simulink model "Non_WindFarm"  (R2024a)
settings: Solver=ode45  StartTime=parSimulacio.ti  StopTime=200  MaxStep=parSimulacio.pas  RelTol=1e-6  AbsTol=1e-6  EnableMultiTasking=on
model workspace (MAT data in the model file):
  tt_vw : Simulink.Parameter (value not decoded)
values from neighbouring files (symbols this model uses):
  L = L'    [Lin_SignalGenerator.m]    (also in Non_ParameterInitialize.m; cal_QR.m = zeros(v, 1); parameters_windFarm2.m)
  nu = size(S, 1)    [Lin_SignalGenerator.m]    (also in Non_ParameterInitialize.m; parameters_windFarm2.m)
  S = zeros(v, v)    [cal_QR.m]
  w0 = [1 -0.00962521549583 0.0254779042049 -0.0160197396127 -0.0156056332727 0.0112137208272 0.0440607583301 -0.0193704893312 -0.0229464276306 -0.00247675309015 0.0285830611299]    [w0.mat]
undefined symbols (not defined in the file or in its folder): parControl, parConvertidor, parGenerador, parGrid, parMecanica, parSimulacio, windspeed
(part 10 of 40)

== system Non_WindFarm/FOM/Wind Farm/Wind Turbine Strings/String6/WT3/WFG ==
  note: input output sign
  note: WE
  note: generator shaft angle
  note: generator speed
  vcqd : Inport
  Bus Continua1 : Subsystem  mask{tempPar=parConvertidor}
      mask prompts: tempPar "Estruc. Parametres"
      mask init:
      | C=tempPar.C;
      | E0=tempPar.E0;
  Clock : Clock
  Constant2 : Constant  Value=10
  Control Electric Generador : Subsystem  mask{tempPar=parControl.Electric.Generador}
      mask prompts: tempPar "Estruc. Parametres"
      mask init: same as Non_WindFarm/FOM/Wind Farm/Wind Turbine Strings/String1/WT1/WFG/Control Electric Generador
  Control Electric Tensio : Subsystem  mask{tempPar=parControl.Electric.BusContinua}
      mask prompts: tempPar "Estruc. Parametres"
      mask init:
      | Kp=tempPar.Kp;
      | Ki=tempPar.Ki;
      | Easterisc=tempPar.Easterisc;
  Control Mecanic : Subsystem  mask{tempPar=parControl.Mecanic}
      mask prompts: tempPar "Escruc. Parametres"
      mask init:
      | %Kp=tempPar.Kp;
      | T=tempPar.T;
      | KCP=tempPar.KCP;
      | omegamn=tempPar.omegamn;
      | Kp=tempPar.Kp;
      | Ki=tempPar.Ki;
  Control de Corrent de Xarxa2 : Subsystem  mask{tempPar=parControl.Electric.BandaXarxa}
      mask prompts: tempPar "Estruc. Parametres"
      mask init:
      | Kp=tempPar.Kp;
      | Ki=tempPar.Ki;
      | Ll=tempPar.Ll;
      | rl=tempPar.rl;
  Filtre de Xarxa1 : Subsystem  mask{tempPar=parConvertidor}
      mask prompts: tempPar "Estruc. Parametres"
      mask init:
      | rl=tempPar.rl;
      | Ll=tempPar.Ll;
  Gain : Gain  Gain=-1
  Maquina Sincrona : Subsystem  mask{tempPar=parGenerador}
      mask prompts: tempPar "Estruct. Parametres"
      mask init:
      | rs=tempPar.rs;
      | Lq=tempPar.Lq;
      | Ld=tempPar.Ld;
      | lambda_m=tempPar.lambda_m;
      | P=tempPar.P;
      | isqd0=tempPar.isqd0;
  Mecanica nolineal i vent : Subsystem  mask{tempPar=parMecanica}
      mask prompts: tempPar "Estruc. Parametres"
      mask init: same as Non_WindFarm/FOM/Wind Farm/Wind Turbine Strings/String1/WT1/WFG/Mecanica nolineal i vent
  Park : Subsystem
  Product1 : Product  Multiplication=Matrix(*)  RndMeth=Zero
  Product4 : Product  Multiplication=Matrix(*)  RndMeth=Zero
  Scope : Scope
  we : Gain  Gain=100*pi
  wind speed : Constant  Value=windspeed.string2
  ilqd : Outport
  wires:
  Mecanica nolineal i vent/1(omega_m) -> Control Electric Generador/4(omega_m), Control Mecanic/1(omega_m), Maquina Sincrona/2(omega_m)
  Mecanica nolineal i vent/2(theta_m) -> Maquina Sincrona/3(theta_m), Control Electric Generador/5(theta_m)
  Maquina Sincrona/2(parell_m) -> Mecanica nolineal i vent/1(parell_m)
  Control de Corrent de Xarxa2/1(vlabc) -> Bus Continua1/2(vlabc), Filtre de Xarxa1/2(vlabc)
  Bus Continua1/1(E) -> Control Electric Tensio/1(E), Control de Corrent de Xarxa2/4(E)
  Maquina Sincrona/1(isabc) -> Bus Continua1/4(isabc), Control Electric Generador/3(isabc)
  Control Electric Generador/1(vscabc) -> Bus Continua1/3(vsabc), Maquina Sincrona/1(vsabc)
  Filtre de Xarxa1/1(ilabc) -> Bus Continua1/1(ilabc), Product1/2, Control de Corrent de Xarxa2/2(ilabc)
  Bus Continua1/2(iDCm) -> Control Electric Tensio/2(IDCm)
  wind speed/1 -> Mecanica nolineal i vent/3(vw)
  Control Electric Tensio/1(iDCla) -> Control de Corrent de Xarxa2/3(iDCla)
  Constant2/1 -> Control Electric Generador/2(Q_sa)
  Control Mecanic/2(theta_a) -> Mecanica nolineal i vent/2(theta_a)
  Park/2(nTthetar) -> Product4/1
  vcqd/1 -> Product4/2
  Product4/1 -> Scope/1, Control de Corrent de Xarxa2/1(vzabc), Filtre de Xarxa1/1(vzabc)
  Park/1(Tthetar) -> Product1/1
  Clock/1 -> we/1
  we/1 -> Park/1(theta_r)
  Gain/1 -> ilqd/1
  Product1/1 -> Gain/1
  Control Mecanic/1(parell_ma) -> Control Electric Generador/1(parell_ma)

== system Non_WindFarm/FOM/Wind Farm/Wind Turbine Strings/String6/WT4/C_cable ==
  note: Vc_cable
  It2 : Inport
  I_in : Inport  Port=2
  I_cable : Inport  Port=3
  Add : Sum  Inputs=++-
  produce Vc_cable : StateSpace  A=[0,-100*pi;100*pi,0]  B=eye(2)/parGrid.WTstring.C_cable  C=eye(2)  D=zeros(2,2)  InitialCondition=sqrt(2)*66000/sqrt(3)*[1;0]
  Vc_cable : Outport
  wires:
  produce Vc_cable/1 -> Vc_cable/1
  Add/1 -> produce Vc_cable/1
  It2/1 -> Add/1
  I_cable/1 -> Add/3
  I_in/1 -> Add/2

== system Non_WindFarm/FOM/Wind Farm/Wind Turbine Strings/String6/WT4/C_filter ==
  note: Vc_filter
  IWF : Inport
  It1 : Inport  Port=2
  Add : Sum  Inputs=+-
  produce Vc_filter : StateSpace  A=[0,-100*pi;100*pi,0]  B=eye(2)/parConvertidor.Cfilt  C=eye(2)  D=zeros(2,2)  InitialCondition=sqrt(2)*970/sqrt(3)*[1;0]
  Vc_filter_qd : Outport
  wires:
  IWF/1 -> Add/1
  It1/1 -> Add/2
  Add/1 -> produce Vc_filter/1
  produce Vc_filter/1 -> Vc_filter_qd/1

== system Non_WindFarm/FOM/Wind Farm/Wind Turbine Strings/String6/WT4/Cable line ==
  V : Inport
  Vc_cable : Inport  Port=2
  1/L_Cable : Gain  Gain=1/parGrid.WTstring.Lcable
  A : Constant  Value=[parGrid.WTstring.rcable,100*pi*parGrid.WTstring.Lcable;-100*pi*parGrid.WTstring.Lcable,parGrid.WTstring.rcable]
  Add : Sum  Inputs=+--
  Integrator : Integrator
  Product6 : Product  Multiplication=Matrix(*)
  I_cable : Outport
  wires:
  Integrator/1 -> Product6/2, I_cable/1
  Vc_cable/1 -> Add/1
  V/1 -> Add/2
  A/1 -> Product6/1
  Product6/1 -> Add/3
  1/L_Cable/1 -> Integrator/1
  Add/1 -> 1/L_Cable/1

== system Non_WindFarm/FOM/Wind Farm/Wind Turbine Strings/String6/WT4/Transformer-complex ==
  note: It1
  note: Vt1
  Vc_filter_qd : Inport
  Vc_cable_qd : Inport  Port=2
  1/(N1N2) : Gain  Gain=1/parGrid.N1N2
  1/(N1N2)1 : Gain  Gain=1/parGrid.N1N2
  1/[Lt+Lt1/(N1N2^2)] : Gain  Gain=1/(parGrid.WTtransf.Lt+parGrid.WTtransf.Lt2/(parGrid.N1N2^2))
  Add4 : Sum  Inputs=-+-
  Integrator2 : Integrator
  Product6 : Product  Multiplication=Matrix(*)
  "[A+A1/(N1N2^2)]" : Constant  Value=[parGrid.WTtransf.rt,100*pi*parGrid.WTtransf.Lt;-100*pi*parGrid.WTtransf.Lt,parGrid.WTtransf.rt]+[parGrid.WTtransf.rt2,100*pi*parGrid.WTtransf.Lt2;-100*pi*parGrid.WTtransf.Lt2,parGrid.WTtransf.rt2]/(parGrid.N1N2^2)
  homopolar sequence : Subsystem  Commented=through
  It1 : Outport
  It2 : Outport  Port=2
  wires:
  Vc_cable_qd/1 -> homopolar sequence/1(Vc_cable_qd)
  Add4/1 -> 1/[Lt+Lt1/(N1N2^2)]/1
  1/(N1N2)/1 -> Add4/1
  Vc_filter_qd/1 -> homopolar sequence/2(Vc_filter_qd)
  Product6/1 -> Add4/3
  Integrator2/1 -> Product6/2, It1/1, 1/(N1N2)1/1
  1/(N1N2)1/1 -> It2/1
  1/[Lt+Lt1/(N1N2^2)]/1 -> Integrator2/1
  homopolar sequence/1(Vc_cable_bar) -> 1/(N1N2)/1
  homopolar sequence/2(Vc_filter_bar) -> Add4/2
  "[A+A1/(N1N2^2)]"/1 -> Product6/1

== system Non_WindFarm/FOM/Wind Farm/Wind Turbine Strings/String6/WT4/WFG ==
  note: input output sign
  note: WE
  note: generator shaft angle
  note: generator speed
  vcqd : Inport
  Bus Continua1 : Subsystem  mask{tempPar=parConvertidor}
      mask prompts: tempPar "Estruc. Parametres"
      mask init:
      | C=tempPar.C;
      | E0=tempPar.E0;
  Clock : Clock
  Constant2 : Constant  Value=10
  Control Electric Generador : Subsystem  mask{tempPar=parControl.Electric.Generador}
      mask prompts: tempPar "Estruc. Parametres"
      mask init: same as Non_WindFarm/FOM/Wind Farm/Wind Turbine Strings/String1/WT1/WFG/Control Electric Generador
  Control Electric Tensio : Subsystem  mask{tempPar=parControl.Electric.BusContinua}
      mask prompts: tempPar "Estruc. Parametres"
      mask init:
      | Kp=tempPar.Kp;
      | Ki=tempPar.Ki;
      | Easterisc=tempPar.Easterisc;
  Control Mecanic : Subsystem  mask{tempPar=parControl.Mecanic}
      mask prompts: tempPar "Escruc. Parametres"
      mask init:
      | %Kp=tempPar.Kp;
      | T=tempPar.T;
      | KCP=tempPar.KCP;
      | omegamn=tempPar.omegamn;
      | Kp=tempPar.Kp;
      | Ki=tempPar.Ki;
  Control de Corrent de Xarxa2 : Subsystem  mask{tempPar=parControl.Electric.BandaXarxa}
      mask prompts: tempPar "Estruc. Parametres"
      mask init:
      | Kp=tempPar.Kp;
      | Ki=tempPar.Ki;
      | Ll=tempPar.Ll;
      | rl=tempPar.rl;
  Filtre de Xarxa1 : Subsystem  mask{tempPar=parConvertidor}
      mask prompts: tempPar "Estruc. Parametres"
      mask init:
      | rl=tempPar.rl;
      | Ll=tempPar.Ll;
  Gain : Gain  Gain=-1
  Maquina Sincrona : Subsystem  mask{tempPar=parGenerador}
      mask prompts: tempPar "Estruct. Parametres"
      mask init:
      | rs=tempPar.rs;
      | Lq=tempPar.Lq;
      | Ld=tempPar.Ld;
      | lambda_m=tempPar.lambda_m;
      | P=tempPar.P;
      | isqd0=tempPar.isqd0;
  Mecanica nolineal i vent : Subsystem  mask{tempPar=parMecanica}
      mask prompts: tempPar "Estruc. Parametres"
      mask init: same as Non_WindFarm/FOM/Wind Farm/Wind Turbine Strings/String1/WT1/WFG/Mecanica nolineal i vent
  Park : Subsystem
  Product1 : Product  Multiplication=Matrix(*)  RndMeth=Zero
  Product4 : Product  Multiplication=Matrix(*)  RndMeth=Zero
  Scope : Scope
  we : Gain  Gain=100*pi
  wind speed : Constant  Value=windspeed.string2
  ilqd : Outport
  wires:
  Mecanica nolineal i vent/1(omega_m) -> Control Electric Generador/4(omega_m), Control Mecanic/1(omega_m), Maquina Sincrona/2(omega_m)
  Mecanica nolineal i vent/2(theta_m) -> Maquina Sincrona/3(theta_m), Control Electric Generador/5(theta_m)
  Maquina Sincrona/2(parell_m) -> Mecanica nolineal i vent/1(parell_m)
  Control de Corrent de Xarxa2/1(vlabc) -> Bus Continua1/2(vlabc), Filtre de Xarxa1/2(vlabc)
  Bus Continua1/1(E) -> Control Electric Tensio/1(E), Control de Corrent de Xarxa2/4(E)
  Maquina Sincrona/1(isabc) -> Bus Continua1/4(isabc), Control Electric Generador/3(isabc)
  Control Electric Generador/1(vscabc) -> Bus Continua1/3(vsabc), Maquina Sincrona/1(vsabc)
  Filtre de Xarxa1/1(ilabc) -> Bus Continua1/1(ilabc), Product1/2, Control de Corrent de Xarxa2/2(ilabc)
  Bus Continua1/2(iDCm) -> Control Electric Tensio/2(IDCm)
  wind speed/1 -> Mecanica nolineal i vent/3(vw)
  Control Electric Tensio/1(iDCla) -> Control de Corrent de Xarxa2/3(iDCla)
  Constant2/1 -> Control Electric Generador/2(Q_sa)
  Control Mecanic/2(theta_a) -> Mecanica nolineal i vent/2(theta_a)
  Park/2(nTthetar) -> Product4/1
  vcqd/1 -> Product4/2
  Product4/1 -> Scope/1, Control de Corrent de Xarxa2/1(vzabc), Filtre de Xarxa1/1(vzabc)
  Park/1(Tthetar) -> Product1/1
  Clock/1 -> we/1
  we/1 -> Park/1(theta_r)
  Gain/1 -> ilqd/1
  Product1/1 -> Gain/1
  Control Mecanic/1(parell_ma) -> Control Electric Generador/1(parell_ma)

== system Non_WindFarm/FOM/Wind Farm/Wind Turbine Strings/String6/WT5/C_cable ==
  note: Vc_cable
  It2 : Inport
  I_in : Inport  Port=2
  I_cable : Inport  Port=3
  Add : Sum  Inputs=++-
  produce Vc_cable : StateSpace  A=[0,-100*pi;100*pi,0]  B=eye(2)/parGrid.WTstring.C_cable  C=eye(2)  D=zeros(2,2)  InitialCondition=sqrt(2)*66000/sqrt(3)*[1;0]
  Vc_cable : Outport
  wires:
  I_in/1 -> Add/2
  I_cable/1 -> Add/3
  It2/1 -> Add/1
  Add/1 -> produce Vc_cable/1
  produce Vc_cable/1 -> Vc_cable/1

== system Non_WindFarm/FOM/Wind Farm/Wind Turbine Strings/String6/WT5/C_filter ==
  note: Vc_filter
  IWF : Inport
  It1 : Inport  Port=2
  Add : Sum  Inputs=+-
  produce Vc_filter : StateSpace  A=[0,-100*pi;100*pi,0]  B=eye(2)/parConvertidor.Cfilt  C=eye(2)  D=zeros(2,2)  InitialCondition=sqrt(2)*970/sqrt(3)*[1;0]
  Vc_filter_qd : Outport
  wires:
  produce Vc_filter/1 -> Vc_filter_qd/1
  Add/1 -> produce Vc_filter/1
  It1/1 -> Add/2
  IWF/1 -> Add/1

== system Non_WindFarm/FOM/Wind Farm/Wind Turbine Strings/String6/WT5/Cable line ==
  V : Inport
  Vc_cable : Inport  Port=2
  1/L_Cable : Gain  Gain=1/parGrid.WTstring.Lcable
  A : Constant  Value=[parGrid.WTstring.rcable,100*pi*parGrid.WTstring.Lcable;-100*pi*parGrid.WTstring.Lcable,parGrid.WTstring.rcable]
  Add : Sum  Inputs=+--
  Integrator : Integrator
  Product6 : Product  Multiplication=Matrix(*)
  I_cable : Outport
  wires:
  Add/1 -> 1/L_Cable/1
  1/L_Cable/1 -> Integrator/1
  Product6/1 -> Add/3
  A/1 -> Product6/1
  V/1 -> Add/2
  Vc_cable/1 -> Add/1
  Integrator/1 -> I_cable/1, Product6/2

== system Non_WindFarm/FOM/Wind Farm/Wind Turbine Strings/String6/WT5/Transformer-complex ==
  note: Vt1
  note: It1
  Vc_filter_qd : Inport
  Vc_cable_qd : Inport  Port=2
  1/(N1N2) : Gain  Gain=1/parGrid.N1N2
  1/(N1N2)1 : Gain  Gain=1/parGrid.N1N2
  1/[Lt+Lt1/(N1N2^2)] : Gain  Gain=1/(parGrid.WTtransf.Lt+parGrid.WTtransf.Lt2/(parGrid.N1N2^2))
  Add4 : Sum  Inputs=-+-
  Integrator2 : Integrator
  Product6 : Product  Multiplication=Matrix(*)
  "[A+A1/(N1N2^2)]" : Constant  Value=[parGrid.WTtransf.rt,100*pi*parGrid.WTtransf.Lt;-100*pi*parGrid.WTtransf.Lt,parGrid.WTtransf.rt]+[parGrid.WTtransf.rt2,100*pi*parGrid.WTtransf.Lt2;-100*pi*parGrid.WTtransf.Lt2,parGrid.WTtransf.rt2]/(parGrid.N1N2^2)
  homopolar sequence : Subsystem  Commented=through
  It1 : Outport
  It2 : Outport  Port=2
  wires:
  "[A+A1/(N1N2^2)]"/1 -> Product6/1
  homopolar sequence/2(Vc_filter_bar) -> Add4/2
  homopolar sequence/1(Vc_cable_bar) -> 1/(N1N2)/1
  1/[Lt+Lt1/(N1N2^2)]/1 -> Integrator2/1
  1/(N1N2)1/1 -> It2/1
  Integrator2/1 -> 1/(N1N2)1/1, It1/1, Product6/2
  Product6/1 -> Add4/3
  Vc_filter_qd/1 -> homopolar sequence/2(Vc_filter_qd)
  1/(N1N2)/1 -> Add4/1
  Add4/1 -> 1/[Lt+Lt1/(N1N2^2)]/1
  Vc_cable_qd/1 -> homopolar sequence/1(Vc_cable_qd)

== system Non_WindFarm/FOM/Wind Farm/Wind Turbine Strings/String6/WT5/WFG ==
  note: input output sign
  note: WE
  note: generator shaft angle
  note: generator speed
  vcqd : Inport
  Bus Continua1 : Subsystem  mask{tempPar=parConvertidor}
      mask prompts: tempPar "Estruc. Parametres"
      mask init:
      | C=tempPar.C;
      | E0=tempPar.E0;
  Clock : Clock
  Constant2 : Constant  Value=10
  Control Electric Generador : Subsystem  mask{tempPar=parControl.Electric.Generador}
      mask prompts: tempPar "Estruc. Parametres"
      mask init: same as Non_WindFarm/FOM/Wind Farm/Wind Turbine Strings/String1/WT1/WFG/Control Electric Generador
  Control Electric Tensio : Subsystem  mask{tempPar=parControl.Electric.BusContinua}
      mask prompts: tempPar "Estruc. Parametres"
      mask init:
      | Kp=tempPar.Kp;
      | Ki=tempPar.Ki;
      | Easterisc=tempPar.Easterisc;
  Control Mecanic : Subsystem  mask{tempPar=parControl.Mecanic}
      mask prompts: tempPar "Escruc. Parametres"
      mask init:
      | %Kp=tempPar.Kp;
      | T=tempPar.T;
      | KCP=tempPar.KCP;
      | omegamn=tempPar.omegamn;
      | Kp=tempPar.Kp;
      | Ki=tempPar.Ki;
  Control de Corrent de Xarxa2 : Subsystem  mask{tempPar=parControl.Electric.BandaXarxa}
      mask prompts: tempPar "Estruc. Parametres"
      mask init:
      | Kp=tempPar.Kp;
      | Ki=tempPar.Ki;
      | Ll=tempPar.Ll;
      | rl=tempPar.rl;
  Filtre de Xarxa1 : Subsystem  mask{tempPar=parConvertidor}
      mask prompts: tempPar "Estruc. Parametres"
      mask init:
      | rl=tempPar.rl;
      | Ll=tempPar.Ll;
  Gain : Gain  Gain=-1
  Maquina Sincrona : Subsystem  mask{tempPar=parGenerador}
      mask prompts: tempPar "Estruct. Parametres"
      mask init:
      | rs=tempPar.rs;
      | Lq=tempPar.Lq;
      | Ld=tempPar.Ld;
      | lambda_m=tempPar.lambda_m;
      | P=tempPar.P;
      | isqd0=tempPar.isqd0;
  Mecanica nolineal i vent : Subsystem  mask{tempPar=parMecanica}
      mask prompts: tempPar "Estruc. Parametres"
      mask init: same as Non_WindFarm/FOM/Wind Farm/Wind Turbine Strings/String1/WT1/WFG/Mecanica nolineal i vent
  Park : Subsystem
  Product1 : Product  Multiplication=Matrix(*)  RndMeth=Zero
  Product4 : Product  Multiplication=Matrix(*)  RndMeth=Zero
  Scope : Scope
  we : Gain  Gain=100*pi
  wind speed : Constant  Value=windspeed.string2
  ilqd : Outport
  wires:
  Mecanica nolineal i vent/1(omega_m) -> Control Electric Generador/4(omega_m), Control Mecanic/1(omega_m), Maquina Sincrona/2(omega_m)
  Mecanica nolineal i vent/2(theta_m) -> Maquina Sincrona/3(theta_m), Control Electric Generador/5(theta_m)
  Maquina Sincrona/2(parell_m) -> Mecanica nolineal i vent/1(parell_m)
  Control de Corrent de Xarxa2/1(vlabc) -> Bus Continua1/2(vlabc), Filtre de Xarxa1/2(vlabc)
  Bus Continua1/1(E) -> Control Electric Tensio/1(E), Control de Corrent de Xarxa2/4(E)
  Maquina Sincrona/1(isabc) -> Bus Continua1/4(isabc), Control Electric Generador/3(isabc)
  Control Electric Generador/1(vscabc) -> Bus Continua1/3(vsabc), Maquina Sincrona/1(vsabc)
  Filtre de Xarxa1/1(ilabc) -> Bus Continua1/1(ilabc), Product1/2, Control de Corrent de Xarxa2/2(ilabc)
  Bus Continua1/2(iDCm) -> Control Electric Tensio/2(IDCm)
  wind speed/1 -> Mecanica nolineal i vent/3(vw)
  Control Electric Tensio/1(iDCla) -> Control de Corrent de Xarxa2/3(iDCla)
  Constant2/1 -> Control Electric Generador/2(Q_sa)
  Control Mecanic/2(theta_a) -> Mecanica nolineal i vent/2(theta_a)
  Park/2(nTthetar) -> Product4/1
  vcqd/1 -> Product4/2
  Product4/1 -> Scope/1, Control de Corrent de Xarxa2/1(vzabc), Filtre de Xarxa1/1(vzabc)
  Park/1(Tthetar) -> Product1/1
  Clock/1 -> we/1
  we/1 -> Park/1(theta_r)
  Gain/1 -> ilqd/1
  Product1/1 -> Gain/1
  Control Mecanic/1(parell_ma) -> Control Electric Generador/1(parell_ma)

== system Non_WindFarm/FOM/Wind Farm/Wind Turbine Strings/String6/WT6/C_cable ==
  note: Vc_cable
  It2 : Inport
  I_in : Inport  Port=2
  I_cable : Inport  Port=3
  Add : Sum  Inputs=++-
  produce Vc_cable : StateSpace  A=[0,-100*pi;100*pi,0]  B=eye(2)/parGrid.WTstring.C_cable  C=eye(2)  D=zeros(2,2)  InitialCondition=sqrt(2)*66000/sqrt(3)*[1;0]
  Vc_cable : Outport
  wires:
  produce Vc_cable/1 -> Vc_cable/1
  Add/1 -> produce Vc_cable/1
  It2/1 -> Add/1
  I_cable/1 -> Add/3
  I_in/1 -> Add/2

== system Non_WindFarm/FOM/Wind Farm/Wind Turbine Strings/String6/WT6/C_filter ==
  note: Vc_filter
  IWF : Inport
  It1 : Inport  Port=2
  Add : Sum  Inputs=+-
  produce Vc_filter : StateSpace  A=[0,-100*pi;100*pi,0]  B=eye(2)/parConvertidor.Cfilt  C=eye(2)  D=zeros(2,2)  InitialCondition=sqrt(2)*970/sqrt(3)*[1;0]
  Vc_filter_qd : Outport
  wires:
  IWF/1 -> Add/1
  It1/1 -> Add/2
  Add/1 -> produce Vc_filter/1
  produce Vc_filter/1 -> Vc_filter_qd/1

== system Non_WindFarm/FOM/Wind Farm/Wind Turbine Strings/String6/WT6/Cable line ==
  V : Inport
  Vc_cable : Inport  Port=2
  1/L_Cable : Gain  Gain=1/parGrid.WTstring.Lcable
  A : Constant  Value=[parGrid.WTstring.rcable,100*pi*parGrid.WTstring.Lcable;-100*pi*parGrid.WTstring.Lcable,parGrid.WTstring.rcable]
  Add : Sum  Inputs=+--
  Integrator : Integrator
  Product6 : Product  Multiplication=Matrix(*)
  I_cable : Outport
  wires:
  Integrator/1 -> Product6/2, I_cable/1
  Vc_cable/1 -> Add/1
  V/1 -> Add/2
  A/1 -> Product6/1
  Product6/1 -> Add/3
  1/L_Cable/1 -> Integrator/1
  Add/1 -> 1/L_Cable/1

== system Non_WindFarm/FOM/Wind Farm/Wind Turbine Strings/String6/WT6/Transformer-complex ==
  note: It1
  note: Vt1
  Vc_filter_qd : Inport
  Vc_cable_qd : Inport  Port=2
  1/(N1N2) : Gain  Gain=1/parGrid.N1N2
  1/(N1N2)1 : Gain  Gain=1/parGrid.N1N2
  1/[Lt+Lt1/(N1N2^2)] : Gain  Gain=1/(parGrid.WTtransf.Lt+parGrid.WTtransf.Lt2/(parGrid.N1N2^2))
  Add4 : Sum  Inputs=-+-
  Integrator2 : Integrator
  Product6 : Product  Multiplication=Matrix(*)
  "[A+A1/(N1N2^2)]" : Constant  Value=[parGrid.WTtransf.rt,100*pi*parGrid.WTtransf.Lt;-100*pi*parGrid.WTtransf.Lt,parGrid.WTtransf.rt]+[parGrid.WTtransf.rt2,100*pi*parGrid.WTtransf.Lt2;-100*pi*parGrid.WTtransf.Lt2,parGrid.WTtransf.rt2]/(parGrid.N1N2^2)
  homopolar sequence : Subsystem  Commented=through
  It1 : Outport
  It2 : Outport  Port=2
  wires:
  Vc_cable_qd/1 -> homopolar sequence/1(Vc_cable_qd)
  Add4/1 -> 1/[Lt+Lt1/(N1N2^2)]/1
  1/(N1N2)/1 -> Add4/1
  Vc_filter_qd/1 -> homopolar sequence/2(Vc_filter_qd)
  Product6/1 -> Add4/3
  Integrator2/1 -> Product6/2, It1/1, 1/(N1N2)1/1
  1/(N1N2)1/1 -> It2/1
  1/[Lt+Lt1/(N1N2^2)]/1 -> Integrator2/1
  homopolar sequence/1(Vc_cable_bar) -> 1/(N1N2)/1
  homopolar sequence/2(Vc_filter_bar) -> Add4/2
  "[A+A1/(N1N2^2)]"/1 -> Product6/1

== system Non_WindFarm/FOM/Wind Farm/Wind Turbine Strings/String6/WT6/WFG ==
  note: input output sign
  note: WE
  note: generator shaft angle
  note: generator speed
  vcqd : Inport
  Bus Continua1 : Subsystem  mask{tempPar=parConvertidor}
      mask prompts: tempPar "Estruc. Parametres"
      mask init:
      | C=tempPar.C;
      | E0=tempPar.E0;
  Clock : Clock
  Constant2 : Constant  Value=10
  Control Electric Generador : Subsystem  mask{tempPar=parControl.Electric.Generador}
      mask prompts: tempPar "Estruc. Parametres"
      mask init: same as Non_WindFarm/FOM/Wind Farm/Wind Turbine Strings/String1/WT1/WFG/Control Electric Generador
  Control Electric Tensio : Subsystem  mask{tempPar=parControl.Electric.BusContinua}
      mask prompts: tempPar "Estruc. Parametres"
      mask init:
      | Kp=tempPar.Kp;
      | Ki=tempPar.Ki;
      | Easterisc=tempPar.Easterisc;
  Control Mecanic : Subsystem  mask{tempPar=parControl.Mecanic}
      mask prompts: tempPar "Escruc. Parametres"
      mask init:
      | %Kp=tempPar.Kp;
      | T=tempPar.T;
      | KCP=tempPar.KCP;
      | omegamn=tempPar.omegamn;
      | Kp=tempPar.Kp;
      | Ki=tempPar.Ki;
  Control de Corrent de Xarxa2 : Subsystem  mask{tempPar=parControl.Electric.BandaXarxa}
      mask prompts: tempPar "Estruc. Parametres"
      mask init:
      | Kp=tempPar.Kp;
      | Ki=tempPar.Ki;
      | Ll=tempPar.Ll;
      | rl=tempPar.rl;
  Filtre de Xarxa1 : Subsystem  mask{tempPar=parConvertidor}
      mask prompts: tempPar "Estruc. Parametres"
      mask init:
      | rl=tempPar.rl;
      | Ll=tempPar.Ll;
  Gain : Gain  Gain=-1
  Maquina Sincrona : Subsystem  mask{tempPar=parGenerador}
      mask prompts: tempPar "Estruct. Parametres"
      mask init:
      | rs=tempPar.rs;
      | Lq=tempPar.Lq;
      | Ld=tempPar.Ld;
      | lambda_m=tempPar.lambda_m;
      | P=tempPar.P;
      | isqd0=tempPar.isqd0;
  Mecanica nolineal i vent : Subsystem  mask{tempPar=parMecanica}
      mask prompts: tempPar "Estruc. Parametres"
      mask init: same as Non_WindFarm/FOM/Wind Farm/Wind Turbine Strings/String1/WT1/WFG/Mecanica nolineal i vent
  Park : Subsystem
  Product1 : Product  Multiplication=Matrix(*)  RndMeth=Zero
  Product4 : Product  Multiplication=Matrix(*)  RndMeth=Zero
  Scope : Scope
  we : Gain  Gain=100*pi
  wind speed : Constant  Value=windspeed.string2
  ilqd : Outport
  wires:
  Mecanica nolineal i vent/1(omega_m) -> Control Electric Generador/4(omega_m), Control Mecanic/1(omega_m), Maquina Sincrona/2(omega_m)
  Mecanica nolineal i vent/2(theta_m) -> Maquina Sincrona/3(theta_m), Control Electric Generador/5(theta_m)
  Maquina Sincrona/2(parell_m) -> Mecanica nolineal i vent/1(parell_m)
  Control de Corrent de Xarxa2/1(vlabc) -> Bus Continua1/2(vlabc), Filtre de Xarxa1/2(vlabc)
  Bus Continua1/1(E) -> Control Electric Tensio/1(E), Control de Corrent de Xarxa2/4(E)
  Maquina Sincrona/1(isabc) -> Bus Continua1/4(isabc), Control Electric Generador/3(isabc)
  Control Electric Generador/1(vscabc) -> Bus Continua1/3(vsabc), Maquina Sincrona/1(vsabc)
  Filtre de Xarxa1/1(ilabc) -> Bus Continua1/1(ilabc), Product1/2, Control de Corrent de Xarxa2/2(ilabc)
  Bus Continua1/2(iDCm) -> Control Electric Tensio/2(IDCm)
  wind speed/1 -> Mecanica nolineal i vent/3(vw)
  Control Electric Tensio/1(iDCla) -> Control de Corrent de Xarxa2/3(iDCla)
  Constant2/1 -> Control Electric Generador/2(Q_sa)
  Control Mecanic/2(theta_a) -> Mecanica nolineal i vent/2(theta_a)
  Park/2(nTthetar) -> Product4/1
  vcqd/1 -> Product4/2
  Product4/1 -> Scope/1, Control de Corrent de Xarxa2/1(vzabc), Filtre de Xarxa1/1(vzabc)
  Park/1(Tthetar) -> Product1/1
  Clock/1 -> we/1
  we/1 -> Park/1(theta_r)
  Gain/1 -> ilqd/1
  Product1/1 -> Gain/1
  Control Mecanic/1(parell_ma) -> Control Electric Generador/1(parell_ma)

== system Non_WindFarm/FOM/Wind Farm/Wind Turbine Strings/String6/WT7/C_cable ==
  note: Vc_cable
  It2 : Inport
  I_in : Inport  Port=2
  I_cable : Inport  Port=3
  Add : Sum  Inputs=++-
  produce Vc_cable : StateSpace  A=[0,-100*pi;100*pi,0]  B=eye(2)/parGrid.WTstring.C_cable  C=eye(2)  D=zeros(2,2)  InitialCondition=sqrt(2)*66000/sqrt(3)*[1;0]
  Vc_cable : Outport
  wires:
  I_in/1 -> Add/2
  I_cable/1 -> Add/3
  It2/1 -> Add/1
  Add/1 -> produce Vc_cable/1
  produce Vc_cable/1 -> Vc_cable/1

== system Non_WindFarm/FOM/Wind Farm/Wind Turbine Strings/String6/WT7/C_filter ==
  note: Vc_filter
  IWF : Inport
  It1 : Inport  Port=2
  Add : Sum  Inputs=+-
  produce Vc_filter : StateSpace  A=[0,-100*pi;100*pi,0]  B=eye(2)/parConvertidor.Cfilt  C=eye(2)  D=zeros(2,2)  InitialCondition=sqrt(2)*970/sqrt(3)*[1;0]
  Vc_filter_qd : Outport
  wires:
  produce Vc_filter/1 -> Vc_filter_qd/1
  Add/1 -> produce Vc_filter/1
  It1/1 -> Add/2
  IWF/1 -> Add/1

== system Non_WindFarm/FOM/Wind Farm/Wind Turbine Strings/String6/WT7/Cable line ==
  V : Inport
  Vc_cable : Inport  Port=2
  1/L_Cable : Gain  Gain=1/parGrid.WTstring.Lcable
  A : Constant  Value=[parGrid.WTstring.rcable,100*pi*parGrid.WTstring.Lcable;-100*pi*parGrid.WTstring.Lcable,parGrid.WTstring.rcable]
  Add : Sum  Inputs=+--
  Integrator : Integrator
  Product6 : Product  Multiplication=Matrix(*)
  I_cable : Outport
  wires:
  Add/1 -> 1/L_Cable/1
  1/L_Cable/1 -> Integrator/1
  Product6/1 -> Add/3
  A/1 -> Product6/1
  V/1 -> Add/2
  Vc_cable/1 -> Add/1
  Integrator/1 -> I_cable/1, Product6/2

== system Non_WindFarm/FOM/Wind Farm/Wind Turbine Strings/String6/WT7/Transformer-complex ==
  note: Vt1
  note: It1
  Vc_filter_qd : Inport
  Vc_cable_qd : Inport  Port=2
  1/(N1N2) : Gain  Gain=1/parGrid.N1N2
  1/(N1N2)1 : Gain  Gain=1/parGrid.N1N2
  1/[Lt+Lt1/(N1N2^2)] : Gain  Gain=1/(parGrid.WTtransf.Lt+parGrid.WTtransf.Lt2/(parGrid.N1N2^2))
  Add4 : Sum  Inputs=-+-
  Integrator2 : Integrator
  Product6 : Product  Multiplication=Matrix(*)
  "[A+A1/(N1N2^2)]" : Constant  Value=[parGrid.WTtransf.rt,100*pi*parGrid.WTtransf.Lt;-100*pi*parGrid.WTtransf.Lt,parGrid.WTtransf.rt]+[parGrid.WTtransf.rt2,100*pi*parGrid.WTtransf.Lt2;-100*pi*parGrid.WTtransf.Lt2,parGrid.WTtransf.rt2]/(parGrid.N1N2^2)
  homopolar sequence : Subsystem  Commented=through
  It1 : Outport
  It2 : Outport  Port=2
  wires:
  "[A+A1/(N1N2^2)]"/1 -> Product6/1
  homopolar sequence/2(Vc_filter_bar) -> Add4/2
  homopolar sequence/1(Vc_cable_bar) -> 1/(N1N2)/1
  1/[Lt+Lt1/(N1N2^2)]/1 -> Integrator2/1
  1/(N1N2)1/1 -> It2/1
  Integrator2/1 -> 1/(N1N2)1/1, It1/1, Product6/2
  Product6/1 -> Add4/3
  Vc_filter_qd/1 -> homopolar sequence/2(Vc_filter_qd)
  1/(N1N2)/1 -> Add4/1
  Add4/1 -> 1/[Lt+Lt1/(N1N2^2)]/1
  Vc_cable_qd/1 -> homopolar sequence/1(Vc_cable_qd)

== system Non_WindFarm/FOM/Wind Farm/Wind Turbine Strings/String6/WT7/WFG ==
  note: input output sign
  note: WE
  note: generator shaft angle
  note: generator speed
  vcqd : Inport
  Bus Continua1 : Subsystem  mask{tempPar=parConvertidor}
      mask prompts: tempPar "Estruc. Parametres"
      mask init:
      | C=tempPar.C;
      | E0=tempPar.E0;
  Clock : Clock
  Constant2 : Constant  Value=10
  Control Electric Generador : Subsystem  mask{tempPar=parControl.Electric.Generador}
      mask prompts: tempPar "Estruc. Parametres"
      mask init: same as Non_WindFarm/FOM/Wind Farm/Wind Turbine Strings/String1/WT1/WFG/Control Electric Generador
  Control Electric Tensio : Subsystem  mask{tempPar=parControl.Electric.BusContinua}
      mask prompts: tempPar "Estruc. Parametres"
      mask init:
      | Kp=tempPar.Kp;
      | Ki=tempPar.Ki;
      | Easterisc=tempPar.Easterisc;
  Control Mecanic : Subsystem  mask{tempPar=parControl.Mecanic}
      mask prompts: tempPar "Escruc. Parametres"
      mask init:
      | %Kp=tempPar.Kp;
      | T=tempPar.T;
      | KCP=tempPar.KCP;
      | omegamn=tempPar.omegamn;
      | Kp=tempPar.Kp;
      | Ki=tempPar.Ki;
  Control de Corrent de Xarxa2 : Subsystem  mask{tempPar=parControl.Electric.BandaXarxa}
      mask prompts: tempPar "Estruc. Parametres"
      mask init:
      | Kp=tempPar.Kp;
      | Ki=tempPar.Ki;
      | Ll=tempPar.Ll;
      | rl=tempPar.rl;
  Filtre de Xarxa1 : Subsystem  mask{tempPar=parConvertidor}
      mask prompts: tempPar "Estruc. Parametres"
      mask init:
      | rl=tempPar.rl;
      | Ll=tempPar.Ll;
  Gain : Gain  Gain=-1
  Maquina Sincrona : Subsystem  mask{tempPar=parGenerador}
      mask prompts: tempPar "Estruct. Parametres"
      mask init:
      | rs=tempPar.rs;
      | Lq=tempPar.Lq;
      | Ld=tempPar.Ld;
      | lambda_m=tempPar.lambda_m;
      | P=tempPar.P;
      | isqd0=tempPar.isqd0;
  Mecanica nolineal i vent : Subsystem  mask{tempPar=parMecanica}
      mask prompts: tempPar "Estruc. Parametres"
      mask init: same as Non_WindFarm/FOM/Wind Farm/Wind Turbine Strings/String1/WT1/WFG/Mecanica nolineal i vent
  Park : Subsystem
  Product1 : Product  Multiplication=Matrix(*)  RndMeth=Zero
  Product4 : Product  Multiplication=Matrix(*)  RndMeth=Zero
  Scope : Scope
  we : Gain  Gain=100*pi
  wind speed : Constant  Value=windspeed.string2
  ilqd : Outport
  wires:
  Mecanica nolineal i vent/1(omega_m) -> Control Electric Generador/4(omega_m), Control Mecanic/1(omega_m), Maquina Sincrona/2(omega_m)
  Mecanica nolineal i vent/2(theta_m) -> Maquina Sincrona/3(theta_m), Control Electric Generador/5(theta_m)
  Maquina Sincrona/2(parell_m) -> Mecanica nolineal i vent/1(parell_m)
  Control de Corrent de Xarxa2/1(vlabc) -> Bus Continua1/2(vlabc), Filtre de Xarxa1/2(vlabc)
  Bus Continua1/1(E) -> Control Electric Tensio/1(E), Control de Corrent de Xarxa2/4(E)
  Maquina Sincrona/1(isabc) -> Bus Continua1/4(isabc), Control Electric Generador/3(isabc)
  Control Electric Generador/1(vscabc) -> Bus Continua1/3(vsabc), Maquina Sincrona/1(vsabc)
  Filtre de Xarxa1/1(ilabc) -> Bus Continua1/1(ilabc), Product1/2, Control de Corrent de Xarxa2/2(ilabc)
  Bus Continua1/2(iDCm) -> Control Electric Tensio/2(IDCm)
  wind speed/1 -> Mecanica nolineal i vent/3(vw)
  Control Electric Tensio/1(iDCla) -> Control de Corrent de Xarxa2/3(iDCla)
  Constant2/1 -> Control Electric Generador/2(Q_sa)
  Control Mecanic/2(theta_a) -> Mecanica nolineal i vent/2(theta_a)
  Park/2(nTthetar) -> Product4/1
  vcqd/1 -> Product4/2
  Product4/1 -> Scope/1, Control de Corrent de Xarxa2/1(vzabc), Filtre de Xarxa1/1(vzabc)
  Park/1(Tthetar) -> Product1/1
  Clock/1 -> we/1
  we/1 -> Park/1(theta_r)
  Gain/1 -> ilqd/1
  Product1/1 -> Gain/1
  Control Mecanic/1(parell_ma) -> Control Electric Generador/1(parell_ma)

== system Non_WindFarm/FOM/Wind Farm/Wind Turbine Strings/String6/WT8/C_cable ==
  note: Vc_cable
  It2 : Inport
  I_in : Inport  Port=2
  I_cable : Inport  Port=3
  Add : Sum  Inputs=++-
  produce Vc_cable : StateSpace  A=[0,-100*pi;100*pi,0]  B=eye(2)/parGrid.WTstring.C_cable  C=eye(2)  D=zeros(2,2)  InitialCondition=sqrt(2)*66000/sqrt(3)*[1;0]
  Vc_cable : Outport
  wires:
  produce Vc_cable/1 -> Vc_cable/1
  Add/1 -> produce Vc_cable/1
  It2/1 -> Add/1
  I_cable/1 -> Add/3
  I_in/1 -> Add/2

== system Non_WindFarm/FOM/Wind Farm/Wind Turbine Strings/String6/WT8/C_filter ==
  note: Vc_filter
  IWF : Inport
  It1 : Inport  Port=2
  Add : Sum  Inputs=+-
  produce Vc_filter : StateSpace  A=[0,-100*pi;100*pi,0]  B=eye(2)/parConvertidor.Cfilt  C=eye(2)  D=zeros(2,2)  InitialCondition=sqrt(2)*970/sqrt(3)*[1;0]
  Vc_filter_qd : Outport
  wires:
  IWF/1 -> Add/1
  It1/1 -> Add/2
  Add/1 -> produce Vc_filter/1
  produce Vc_filter/1 -> Vc_filter_qd/1

== system Non_WindFarm/FOM/Wind Farm/Wind Turbine Strings/String6/WT8/Cable line ==
  V : Inport
  Vc_cable : Inport  Port=2
  1/L_Cable : Gain  Gain=1/parGrid.WTstring.Lcable
  A : Constant  Value=[parGrid.WTstring.rcable,100*pi*parGrid.WTstring.Lcable;-100*pi*parGrid.WTstring.Lcable,parGrid.WTstring.rcable]
  Add : Sum  Inputs=+--
  Integrator : Integrator
  Product6 : Product  Multiplication=Matrix(*)
  I_cable : Outport
  wires:
  Integrator/1 -> Product6/2, I_cable/1
  Vc_cable/1 -> Add/1
  V/1 -> Add/2
  A/1 -> Product6/1
  Product6/1 -> Add/3
  1/L_Cable/1 -> Integrator/1
  Add/1 -> 1/L_Cable/1

== system Non_WindFarm/FOM/Wind Farm/Wind Turbine Strings/String6/WT8/Transformer-complex ==
  note: It1
  note: Vt1
  Vc_filter_qd : Inport
  Vc_cable_qd : Inport  Port=2
  1/(N1N2) : Gain  Gain=1/parGrid.N1N2
  1/(N1N2)1 : Gain  Gain=1/parGrid.N1N2
  1/[Lt+Lt1/(N1N2^2)] : Gain  Gain=1/(parGrid.WTtransf.Lt+parGrid.WTtransf.Lt2/(parGrid.N1N2^2))
  Add4 : Sum  Inputs=-+-
  Integrator2 : Integrator
  Product6 : Product  Multiplication=Matrix(*)
  "[A+A1/(N1N2^2)]" : Constant  Value=[parGrid.WTtransf.rt,100*pi*parGrid.WTtransf.Lt;-100*pi*parGrid.WTtransf.Lt,parGrid.WTtransf.rt]+[parGrid.WTtransf.rt2,100*pi*parGrid.WTtransf.Lt2;-100*pi*parGrid.WTtransf.Lt2,parGrid.WTtransf.rt2]/(parGrid.N1N2^2)
  homopolar sequence : Subsystem  Commented=through
  It1 : Outport
  It2 : Outport  Port=2
  wires:
  Vc_cable_qd/1 -> homopolar sequence/1(Vc_cable_qd)
  Add4/1 -> 1/[Lt+Lt1/(N1N2^2)]/1
  1/(N1N2)/1 -> Add4/1
  Vc_filter_qd/1 -> homopolar sequence/2(Vc_filter_qd)
  Product6/1 -> Add4/3
  Integrator2/1 -> Product6/2, It1/1, 1/(N1N2)1/1
  1/(N1N2)1/1 -> It2/1
  1/[Lt+Lt1/(N1N2^2)]/1 -> Integrator2/1
  homopolar sequence/1(Vc_cable_bar) -> 1/(N1N2)/1
  homopolar sequence/2(Vc_filter_bar) -> Add4/2
  "[A+A1/(N1N2^2)]"/1 -> Product6/1

== system Non_WindFarm/FOM/Wind Farm/Wind Turbine Strings/String6/WT8/WFG ==
  note: input output sign
  note: WE
  note: generator shaft angle
  note: generator speed
  vcqd : Inport
  Bus Continua1 : Subsystem  mask{tempPar=parConvertidor}
      mask prompts: tempPar "Estruc. Parametres"
      mask init:
      | C=tempPar.C;
      | E0=tempPar.E0;
  Clock : Clock
  Constant2 : Constant  Value=10
  Control Electric Generador : Subsystem  mask{tempPar=parControl.Electric.Generador}
      mask prompts: tempPar "Estruc. Parametres"
      mask init: same as Non_WindFarm/FOM/Wind Farm/Wind Turbine Strings/String1/WT1/WFG/Control Electric Generador
  Control Electric Tensio : Subsystem  mask{tempPar=parControl.Electric.BusContinua}
      mask prompts: tempPar "Estruc. Parametres"
      mask init:
      | Kp=tempPar.Kp;
      | Ki=tempPar.Ki;
      | Easterisc=tempPar.Easterisc;
  Control Mecanic : Subsystem  mask{tempPar=parControl.Mecanic}
      mask prompts: tempPar "Escruc. Parametres"
      mask init:
      | %Kp=tempPar.Kp;
      | T=tempPar.T;
      | KCP=tempPar.KCP;
      | omegamn=tempPar.omegamn;
      | Kp=tempPar.Kp;
      | Ki=tempPar.Ki;
  Control de Corrent de Xarxa2 : Subsystem  mask{tempPar=parControl.Electric.BandaXarxa}
      mask prompts: tempPar "Estruc. Parametres"
      mask init:
      | Kp=tempPar.Kp;
      | Ki=tempPar.Ki;
      | Ll=tempPar.Ll;
      | rl=tempPar.rl;
  Filtre de Xarxa1 : Subsystem  mask{tempPar=parConvertidor}
      mask prompts: tempPar "Estruc. Parametres"
      mask init:
      | rl=tempPar.rl;
      | Ll=tempPar.Ll;
  Gain : Gain  Gain=-1
  Maquina Sincrona : Subsystem  mask{tempPar=parGenerador}
      mask prompts: tempPar "Estruct. Parametres"
      mask init:
      | rs=tempPar.rs;
      | Lq=tempPar.Lq;
      | Ld=tempPar.Ld;
      | lambda_m=tempPar.lambda_m;
      | P=tempPar.P;
      | isqd0=tempPar.isqd0;
  Mecanica nolineal i vent : Subsystem  mask{tempPar=parMecanica}
      mask prompts: tempPar "Estruc. Parametres"
      mask init: same as Non_WindFarm/FOM/Wind Farm/Wind Turbine Strings/String1/WT1/WFG/Mecanica nolineal i vent
  Park : Subsystem
  Product1 : Product  Multiplication=Matrix(*)  RndMeth=Zero
  Product4 : Product  Multiplication=Matrix(*)  RndMeth=Zero
  Scope : Scope
  we : Gain  Gain=100*pi
  wind speed : Constant  Value=windspeed.string2
  ilqd : Outport
  wires:
  Mecanica nolineal i vent/1(omega_m) -> Control Electric Generador/4(omega_m), Control Mecanic/1(omega_m), Maquina Sincrona/2(omega_m)
  Mecanica nolineal i vent/2(theta_m) -> Maquina Sincrona/3(theta_m), Control Electric Generador/5(theta_m)
  Maquina Sincrona/2(parell_m) -> Mecanica nolineal i vent/1(parell_m)
  Control de Corrent de Xarxa2/1(vlabc) -> Bus Continua1/2(vlabc), Filtre de Xarxa1/2(vlabc)
  Bus Continua1/1(E) -> Control Electric Tensio/1(E), Control de Corrent de Xarxa2/4(E)
  Maquina Sincrona/1(isabc) -> Bus Continua1/4(isabc), Control Electric Generador/3(isabc)
  Control Electric Generador/1(vscabc) -> Bus Continua1/3(vsabc), Maquina Sincrona/1(vsabc)
  Filtre de Xarxa1/1(ilabc) -> Bus Continua1/1(ilabc), Product1/2, Control de Corrent de Xarxa2/2(ilabc)
  Bus Continua1/2(iDCm) -> Control Electric Tensio/2(IDCm)
  wind speed/1 -> Mecanica nolineal i vent/3(vw)
  Control Electric Tensio/1(iDCla) -> Control de Corrent de Xarxa2/3(iDCla)
  Constant2/1 -> Control Electric Generador/2(Q_sa)
  Control Mecanic/2(theta_a) -> Mecanica nolineal i vent/2(theta_a)
  Park/2(nTthetar) -> Product4/1
  vcqd/1 -> Product4/2
  Product4/1 -> Scope/1, Control de Corrent de Xarxa2/1(vzabc), Filtre de Xarxa1/1(vzabc)
  Park/1(Tthetar) -> Product1/1
  Clock/1 -> we/1
  we/1 -> Park/1(theta_r)
  Gain/1 -> ilqd/1
  Product1/1 -> Gain/1
  Control Mecanic/1(parell_ma) -> Control Electric Generador/1(parell_ma)

== system Non_WindFarm/FOM/Wind Farm/Wind Turbine Strings/String6/WT9/C_cable ==
  note: Vc_cable
  It2 : Inport
  I_in : Inport  Port=2
  I_cable : Inport  Port=3
  Add : Sum  Inputs=++-
  produce Vc_cable : StateSpace  A=[0,-100*pi;100*pi,0]  B=eye(2)/parGrid.WTstring.C_cable  C=eye(2)  D=zeros(2,2)  InitialCondition=sqrt(2)*66000/sqrt(3)*[1;0]
  Vc_cable : Outport
  wires:
  I_in/1 -> Add/2
  I_cable/1 -> Add/3
  It2/1 -> Add/1
  Add/1 -> produce Vc_cable/1
  produce Vc_cable/1 -> Vc_cable/1

== system Non_WindFarm/FOM/Wind Farm/Wind Turbine Strings/String6/WT9/C_filter ==
  note: Vc_filter
  IWF : Inport
  It1 : Inport  Port=2
  Add : Sum  Inputs=+-
  produce Vc_filter : StateSpace  A=[0,-100*pi;100*pi,0]  B=eye(2)/parConvertidor.Cfilt  C=eye(2)  D=zeros(2,2)  InitialCondition=sqrt(2)*970/sqrt(3)*[1;0]
  Vc_filter_qd : Outport
  wires:
  produce Vc_filter/1 -> Vc_filter_qd/1
  Add/1 -> produce Vc_filter/1
  It1/1 -> Add/2
  IWF/1 -> Add/1

== system Non_WindFarm/FOM/Wind Farm/Wind Turbine Strings/String6/WT9/Cable line ==
  V : Inport
  Vc_cable : Inport  Port=2
  1/L_Cable : Gain  Gain=1/parGrid.WTstring.Lcable
  A : Constant  Value=[parGrid.WTstring.rcable,100*pi*parGrid.WTstring.Lcable;-100*pi*parGrid.WTstring.Lcable,parGrid.WTstring.rcable]
  Add : Sum  Inputs=+--
  Integrator : Integrator
  Product6 : Product  Multiplication=Matrix(*)
  I_cable : Outport
  wires:
  Add/1 -> 1/L_Cable/1
  1/L_Cable/1 -> Integrator/1
  Product6/1 -> Add/3
  A/1 -> Product6/1
  V/1 -> Add/2
  Vc_cable/1 -> Add/1
  Integrator/1 -> I_cable/1, Product6/2

== system Non_WindFarm/FOM/Wind Farm/Wind Turbine Strings/String6/WT9/Transformer-complex ==
  note: Vt1
  note: It1
  Vc_filter_qd : Inport
  Vc_cable_qd : Inport  Port=2
  1/(N1N2) : Gain  Gain=1/parGrid.N1N2
  1/(N1N2)1 : Gain  Gain=1/parGrid.N1N2
  1/[Lt+Lt1/(N1N2^2)] : Gain  Gain=1/(parGrid.WTtransf.Lt+parGrid.WTtransf.Lt2/(parGrid.N1N2^2))
  Add4 : Sum  Inputs=-+-
  Integrator2 : Integrator
  Product6 : Product  Multiplication=Matrix(*)
  "[A+A1/(N1N2^2)]" : Constant  Value=[parGrid.WTtransf.rt,100*pi*parGrid.WTtransf.Lt;-100*pi*parGrid.WTtransf.Lt,parGrid.WTtransf.rt]+[parGrid.WTtransf.rt2,100*pi*parGrid.WTtransf.Lt2;-100*pi*parGrid.WTtransf.Lt2,parGrid.WTtransf.rt2]/(parGrid.N1N2^2)
  homopolar sequence : Subsystem  Commented=through
  It1 : Outport
  It2 : Outport  Port=2
  wires:
  "[A+A1/(N1N2^2)]"/1 -> Product6/1
  homopolar sequence/2(Vc_filter_bar) -> Add4/2
  homopolar sequence/1(Vc_cable_bar) -> 1/(N1N2)/1
  1/[Lt+Lt1/(N1N2^2)]/1 -> Integrator2/1
  1/(N1N2)1/1 -> It2/1
  Integrator2/1 -> 1/(N1N2)1/1, It1/1, Product6/2
  Product6/1 -> Add4/3
  Vc_filter_qd/1 -> homopolar sequence/2(Vc_filter_qd)
  1/(N1N2)/1 -> Add4/1
  Add4/1 -> 1/[Lt+Lt1/(N1N2^2)]/1
  Vc_cable_qd/1 -> homopolar sequence/1(Vc_cable_qd)

== system Non_WindFarm/FOM/Wind Farm/Wind Turbine Strings/String6/WT9/WFG ==
  note: input output sign
  note: WE
  note: generator shaft angle
  note: generator speed
  vcqd : Inport
  Bus Continua1 : Subsystem  mask{tempPar=parConvertidor}
      mask prompts: tempPar "Estruc. Parametres"
      mask init:
      | C=tempPar.C;
      | E0=tempPar.E0;
  Clock : Clock
  Constant2 : Constant  Value=10
  Control Electric Generador : Subsystem  mask{tempPar=parControl.Electric.Generador}
      mask prompts: tempPar "Estruc. Parametres"
      mask init: same as Non_WindFarm/FOM/Wind Farm/Wind Turbine Strings/String1/WT1/WFG/Control Electric Generador
  Control Electric Tensio : Subsystem  mask{tempPar=parControl.Electric.BusContinua}
      mask prompts: tempPar "Estruc. Parametres"
      mask init:
      | Kp=tempPar.Kp;
      | Ki=tempPar.Ki;
      | Easterisc=tempPar.Easterisc;
  Control Mecanic : Subsystem  mask{tempPar=parControl.Mecanic}
      mask prompts: tempPar "Escruc. Parametres"
      mask init:
      | %Kp=tempPar.Kp;
      | T=tempPar.T;
      | KCP=tempPar.KCP;
      | omegamn=tempPar.omegamn;
      | Kp=tempPar.Kp;
      | Ki=tempPar.Ki;
  Control de Corrent de Xarxa2 : Subsystem  mask{tempPar=parControl.Electric.BandaXarxa}
      mask prompts: tempPar "Estruc. Parametres"
      mask init:
      | Kp=tempPar.Kp;
      | Ki=tempPar.Ki;
      | Ll=tempPar.Ll;
      | rl=tempPar.rl;
  Filtre de Xarxa1 : Subsystem  mask{tempPar=parConvertidor}
      mask prompts: tempPar "Estruc. Parametres"
      mask init:
      | rl=tempPar.rl;
      | Ll=tempPar.Ll;
  Gain : Gain  Gain=-1
  Maquina Sincrona : Subsystem  mask{tempPar=parGenerador}
      mask prompts: tempPar "Estruct. Parametres"
      mask init:
      | rs=tempPar.rs;
      | Lq=tempPar.Lq;
      | Ld=tempPar.Ld;
      | lambda_m=tempPar.lambda_m;
      | P=tempPar.P;
      | isqd0=tempPar.isqd0;
  Mecanica nolineal i vent : Subsystem  mask{tempPar=parMecanica}
      mask prompts: tempPar "Estruc. Parametres"
      mask init: same as Non_WindFarm/FOM/Wind Farm/Wind Turbine Strings/String1/WT1/WFG/Mecanica nolineal i vent
  Park : Subsystem
  Product1 : Product  Multiplication=Matrix(*)  RndMeth=Zero
  Product4 : Product  Multiplication=Matrix(*)  RndMeth=Zero
  Scope : Scope
  we : Gain  Gain=100*pi
  wind speed : Constant  Value=windspeed.string2
  ilqd : Outport
  wires:
  Mecanica nolineal i vent/1(omega_m) -> Control Electric Generador/4(omega_m), Control Mecanic/1(omega_m), Maquina Sincrona/2(omega_m)
  Mecanica nolineal i vent/2(theta_m) -> Maquina Sincrona/3(theta_m), Control Electric Generador/5(theta_m)
  Maquina Sincrona/2(parell_m) -> Mecanica nolineal i vent/1(parell_m)
  Control de Corrent de Xarxa2/1(vlabc) -> Bus Continua1/2(vlabc), Filtre de Xarxa1/2(vlabc)
  Bus Continua1/1(E) -> Control Electric Tensio/1(E), Control de Corrent de Xarxa2/4(E)
  Maquina Sincrona/1(isabc) -> Bus Continua1/4(isabc), Control Electric Generador/3(isabc)
  Control Electric Generador/1(vscabc) -> Bus Continua1/3(vsabc), Maquina Sincrona/1(vsabc)
  Filtre de Xarxa1/1(ilabc) -> Bus Continua1/1(ilabc), Product1/2, Control de Corrent de Xarxa2/2(ilabc)
  Bus Continua1/2(iDCm) -> Control Electric Tensio/2(IDCm)
  wind speed/1 -> Mecanica nolineal i vent/3(vw)
  Control Electric Tensio/1(iDCla) -> Control de Corrent de Xarxa2/3(iDCla)
  Constant2/1 -> Control Electric Generador/2(Q_sa)
  Control Mecanic/2(theta_a) -> Mecanica nolineal i vent/2(theta_a)
  Park/2(nTthetar) -> Product4/1
  vcqd/1 -> Product4/2
  Product4/1 -> Scope/1, Control de Corrent de Xarxa2/1(vzabc), Filtre de Xarxa1/1(vzabc)
  Park/1(Tthetar) -> Product1/1
  Clock/1 -> we/1
  we/1 -> Park/1(theta_r)
  Gain/1 -> ilqd/1
  Product1/1 -> Gain/1
  Control Mecanic/1(parell_ma) -> Control Electric Generador/1(parell_ma)

== system Non_WindFarm/FOM/Wind Farm/Wind Turbine Strings/String1/WT1/Transformer-complex/homopolar sequence ==
  note: Vc_filter_qd_bar
  note: Vc_filter_abc_bar
  note: WE
  note: Vc_cable_qd_bar
  note: Vc_cable_abc_bar
  Vc_cable_qd : Inport
  Vc_filter_qd : Inport  Port=2
  Clock : Clock
  Park : Subsystem
  Product{3..5,7} (4 alike) : Product  Multiplication=Matrix(*)  RndMeth=Zero
  homopolar sequence 1 : Subsystem
  homopolar sequence 2 : Subsystem
  we : Gain  Gain=100*pi
  Vc_cable_bar : Outport
  Vc_filter_bar : Outport  Port=2
  wires:
  Product7/1 -> Vc_cable_bar/1
  Product3/1 -> homopolar sequence 1/1(v)
  Vc_filter_qd/1 -> Product3/2
  Vc_cable_qd/1 -> Product4/2
  Product5/1 -> Vc_filter_bar/1
  we/1 -> Park/1(theta_r)
  Clock/1 -> we/1
  homopolar sequence 1/1(v_bar) -> Product5/2
  homopolar sequence 2/1(v_bar) -> Product7/2
  Product4/1 -> homopolar sequence 2/1(v)
  Park/1(Tthetar) -> Product7/1, Product5/1
  Park/2(nTthetar) -> Product4/1, Product3/1

== system Non_WindFarm/FOM/Wind Farm/Wind Turbine Strings/String1/WT1/WFG/Bus Continua1 ==
  note: E=-V_DC?
  note: V_DC/R_DC ?
  note: Eq 5.2-5.5
  ilabc : Inport
  vlabc : Inport  Port=2
  vsabc : Inport  Port=3
  isabc : Inport  Port=4
  Add : Sum  Inputs=+++
  Add1 : Sum  Inputs=+++
  Demux : Demux  Outputs=3
  Demux1 : Demux  Outputs=3
  Divide : Product  Inputs=*/
  Divide1 : Product  Inputs=*/
  Gain : Gain  Gain=1/C
  Integrator : Integrator  InitialCondition=E0  LowerSaturationLimit=10
  Product : Product  RndMeth=Zero
  Product1 : Product  RndMeth=Zero
  Saturation : Saturate  UpperLimit=inf  LowerLimit=1e-3
  Sum : Sum  Inputs=|+-
  To Workspace7 : ToWorkspace  VariableName=capiDCl  SampleTime=parSimulacio.captura.Tmostreig
      settings: Decimation=parSimulacio.captura.Delmat
  E : Outport
  iDCm : Outport  Port=2
  wires:
  Divide1/1 -> To Workspace7/1, Sum/1
  Add1/1 -> Divide1/1
  vlabc/1 -> Product1/2
  Demux1/1 -> Add1/1
  Demux1/2 -> Add1/2
  Product1/1 -> Demux1/1
  ilabc/1 -> Product1/1
  Demux1/3 -> Add1/3
  Integrator/1 -> E/1, Saturation/1
  Saturation/1 -> Divide1/2, Divide/2
  Divide/1 -> Sum/2, iDCm/1
  Add/1 -> Divide/1
  isabc/1 -> Product/2
  vsabc/1 -> Product/1
  Gain/1 -> Integrator/1
  Sum/1 -> Gain/1
  Demux/3 -> Add/3
  Demux/2 -> Add/2
  Demux/1 -> Add/1
  Product/1 -> Demux/1

== system Non_WindFarm/FOM/Wind Farm/Wind Turbine Strings/String1/WT1/WFG/Control Electric Generador ==
  note: voltage source converter
  note: Vs_qd_hat(control output)
  note: 10.14
  note: Vs_qd
  note: 4.25
  note: continuous PI
  note: 4.22
  note: 4.22
  parell_ma : Inport
  Q_sa : Inport  Port=2
  isabc : Inport  Port=3
  omega_m : Inport  Port=4
  theta_m : Inport  Port=5
  Constant1 : Constant  Value=0
  Constant2 : Constant  Value=0
  Constant5 : Constant  Value=0
  Divide : Product  Inputs=*/
  Gain : Gain  Gain=-Lq
  Gain1 : Gain  Gain=Ld
  Gain2 : Gain  Gain=lambda_m
  Gain3 : Gain  Gain=P
  Gain4 : Gain  Gain=2/(3*P)
  Gain5 : Gain  Gain=1/lambda_m
  Gain6 : Gain  Gain=2/3
  Gain7 : Gain  Gain=P
  Gain8 : Gain  Gain=1/lambda_m
  Matrix Concatenate : Concatenate  Mode=Multidimensional array  ConcatenateDimension=2
  Memory : Memory  Commented=through
  Mux{,1..3} (4 alike) : Mux  Inputs=2
  PI : Subsystem
  Park : Subsystem
  Product1 : Product  Multiplication=Matrix(*)  RndMeth=Zero
  Product2 : Product  Multiplication=Matrix(*)  RndMeth=Zero
  Product4 : Product  Multiplication=Matrix(*)  RndMeth=Zero
  Sat inf : Subsystem
  Sum : Sum  Inputs=|++
  Sum1 : Sum  Inputs=|+-
  Sum2 : Sum  Inputs=++|
  To Workspace : ToWorkspace  VariableName=capisqd  SampleTime=parSimulacio.captura.Tmostreig
      settings: Decimation=parSimulacio.captura.Delmat
  To Workspace1 : ToWorkspace  VariableName=capisqda  SampleTime=parSimulacio.captura.Tmostreig
      settings: Decimation=parSimulacio.captura.Delmat
  To Workspace2 : ToWorkspace  VariableName=capvscqd  SampleTime=parSimulacio.captura.Tmostreig
      settings: Decimation=parSimulacio.captura.Delmat
  To Workspace3 : ToWorkspace  VariableName=capvscabc  SampleTime=parSimulacio.captura.Tmostreig
      settings: Decimation=parSimulacio.captura.Delmat
  vscabc : Outport
  wires:
  Gain7/1 -> Park/1(theta_r)
  Park/1(Tthetar) -> Product4/1
  Constant2/1 -> Mux/1
  Gain1/1 -> Mux/2
  Gain/1 -> Mux1/1
  Constant1/1 -> Mux1/2
  Mux/1 -> Matrix Concatenate/1
  Mux1/1 -> Matrix Concatenate/2
  Matrix Concatenate/1 -> Product1/1
  Product4/1 -> Product1/2, Sum1/2, To Workspace/1
  omega_m/1 -> Gain3/1
  Product1/1 -> Sum/2
  Sum2/1 -> Product2/2, To Workspace2/1
  Sum1/1 -> PI/1(e)
  PI/1(u) -> Sum2/2
  Mux2/1 -> Sum1/1, To Workspace1/1
  theta_m/1 -> Gain7/1
  isabc/1 -> Product4/2
  Product2/1 -> Memory/1
  Gain3/1 -> Gain1/1, Gain2/1, Gain/1, Sat inf/1(in)
  Mux3/1 -> Sum/1
  Gain2/1 -> Mux3/1
  Constant5/1 -> Mux3/2
  Park/2(nTthetar) -> Product2/1
  Sum/1 -> Sum2/1
  Gain4/1 -> Mux2/1
  Gain5/1 -> Gain4/1
  Gain8/1 -> Gain6/1
  Q_sa/1 -> Divide/1
  Memory/1 -> vscabc/1, To Workspace3/1
  parell_ma/1 -> Gain5/1
  Sat inf/1(out) -> Divide/2
  Divide/1 -> Gain8/1
  Gain6/1 -> Mux2/2
